simulink model "bai3a"  (R2014a)
settings: Solver=ode45  SolverMode=SingleTasking  StartTime=0.0  StopTime=1000  RelTol=1e-3
libraries: simulink x1
settings Model: CovMetricSettings=dwe  CovHtmlReporting=off  covSaveCumulativeToWorkspaceVar=off  CovSaveSingleToWorkspaceVar=off  CovExternalEMLEnable=on  CovSFcnEnable=on  Creator=DELL  LastModifiedBy=DELL
settings DataIOCC: LimitDataPoints=off  SaveFormat=StructureWithTime  ReturnWorkspaceOutputs=on
settings DebuggingCC: MergeDetectMultiDrivingBlocksExec=error  SolverPrmCheckMsg=none  FrameProcessingCompatibilityMsg=error  SFUnexpectedBacktrackingDiag=error  SFNoUnconditionalDefaultTransitionDiag=error
settings HardwareCC: ProdBitPerPointer=64  ProdLargestAtomicFloat=Float  ProdIntDivRoundTo=Zero  ProdEndianess=LittleEndian  ProdHWDeviceType=Specified
settings ModelReferenceCC: PropagateSignalLabelsOutOfModel=on
settings SFSimCC: SimUseLocalCustomCode=on
settings RTWCC: RTWUseLocalCustomCode=on
settings GRTTargetCC: TargetLangStandard=C99 (ISO)  GeneratePreprocessorConditionals=Use local settings

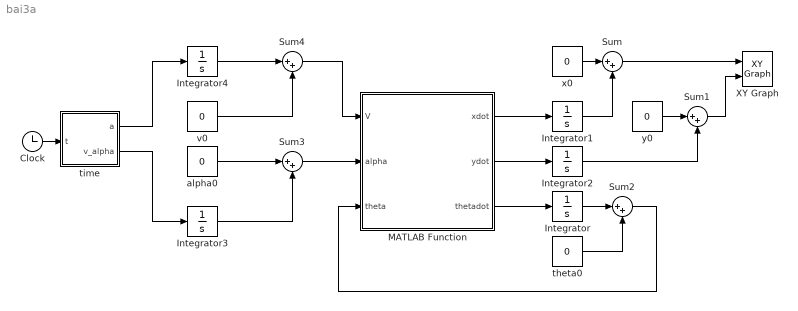
== system bai3a ==
  Clock : Clock
      settings: Decimation=2
  Integrator{,1..4} (5 alike) : Integrator
  MATLAB Function : MATLAB Function  TreatAsAtomicUnit=on
      settings: PermitHierarchicalResolution=ParametersOnly
  Sum{,1..4} (5 alike) : Sum  Inputs=|++
  XY Graph : simulink/Sinks/XY Graph  xmin=-10  xmax=30  ymin=-20  ymax=30  st=-1
  alpha0 : Constant  Value=0
  "theta0 " : Constant  Value=0
  time : MATLAB Function  TreatAsAtomicUnit=on
      settings: PermitHierarchicalResolution=ParametersOnly
  "v0 " : Constant  Value=0
  "x0 " : Constant  Value=0
  y0 : Constant  Value=0
  wires:
  "v0 "/1 -> Sum4/2
  MATLAB Function/3(thetadot) -> Integrator/1
  MATLAB Function/2(ydot) -> Integrator2/1
  MATLAB Function/1(xdot) -> Integrator1/1
  Integrator/1 -> Sum2/1
  "theta0 "/1 -> Sum2/2
  "x0 "/1 -> Sum/1
  Integrator1/1 -> Sum/2
  Sum/1 -> XY Graph/1
  Integrator2/1 -> Sum1/2
  y0/1 -> Sum1/1
  Sum1/1 -> XY Graph/2
  Sum2/1 -> MATLAB Function/3(theta)
  time/2(v_alpha) -> Integrator3/1
  Integrator3/1 -> Sum3/2
  Sum3/1 -> MATLAB Function/2(alpha)
  time/1(a) -> Integrator4/1
  Integrator4/1 -> Sum4/1
  Sum4/1 -> MATLAB Function/1(V)
  Clock/1 -> time/1(t)
  alpha0/1 -> Sum3/1

== matlab function bai3a/time ==
  data: t input; a output; v_alpha output
function [a, v_alpha] = fcn(t)

a = 0; %gia toc
v_alpha = 0; %van toc goc lai
d = sqrt(5); %chieu dai truc co so
alpha = atan2(d,4); % tinh toan goc alpha

t1 = 20/3; %thoi gian di 10m
t2 = alpha/0.3; %thoi gian de xe quay goc alpha
t3 = sqrt(pi*80/9);%thoi gian di nua duong tron R = 4m

%di 10m dau tien voi gia toc a = 0.45
if t < t1
    a = 0.45;
    v_alpha = 0;
%di 10m sau voi gia toc a = -0.45
elseif t >= t1 && t < t1*2
    a = -0.45;
    v_alpha = 0;
%xoay goc lai
elseif t >= t1*2 && t < t1*2 + t2
    a = 0;
    v_alpha = -0.3;
%di nua duong tron voi a = 0.45
elseif t >= t1*2 + t2  && t < t1*2 + t2 + t3
    a = 0.45;
    v_alpha = 0;
%di nua duong tron voi a = -0.45
elseif t >= t1*2 + t2 + t3  && t < t1*2 + t2 + t3*2
    a = -0.45;
    v_alpha = 0;
%xoay goc lai
elseif t >= t1*2 + t2 + t3*2   && t < t1*2 + t2*2 + t3*2 +0.0886 
    a = 0;
    v_alpha = 0.3;
%di 10m voi gia toc a = 0.45
elseif t >= t1*2 + t2*2 + t3*2 + 0.0886    && t < t1*3 + t2*2 + t3*2+ 0.2962515
    a = 0.45;
    v_alpha = 0;
%di 10m gia toc a = -0.45
elseif t >= t1*3 + t2*2 + t3*2+ 0.2962515  && t < t1*4 + t2*2 + t3*2
    a = -0.45;
    v_alpha = 0; 

end

== matlab function bai3a/MATLAB Function ==
  data: V input; xdot output; alpha input; theta input; ydot output; thetadot output
function [xdot,ydot,thetadot]= fcn(V,alpha,theta)
%chieu dai truc co so
d = sqrt(2.5+0.1*25);
%gioi han goc alpha max
if abs(alpha) > pi/4
    alpha = pi/4*sign(alpha);
end
%gioi han van toc max
if V > 1.5 + 0.03*25
    V = 1.5 + 0.03*25;
elseif V < 0
    V = 0;
end
%phuong trinh chuyen dong
%TH1
% xdot = V*cos(alpha)*cos(theta);
% ydot = V*cos(alpha)*sin(theta);
% thetadot = V*sin(alpha)/d;

%TH2
xdot = V*cos(theta);
ydot = V*sin(theta);
thetadot = V*tan(alpha)/d;
